simulink model "AQLRL"  (R2023b)
settings: Solver=FixedStepAuto  StartTime=0.0  StopTime=74.975  FixedStep=0.025  RelTol=1e-3
model workspace (MAT data in the model file):
  A = Simulink.Parameter
  A.Value = [1  0.025  0  0  0  0; 0  1  0  0  0  0; 0  0  1  0.025  0  0; 0  0  0  1  0  0; 0  0  0  0  1  0.025; 0  0  0  0  0  1]
  A.DataType = 'auto'
  A.Complexity = 'real'
  A.Dimensions = [6 6]
  Aag = Simulink.Parameter
  Aag.Value = [1  0.025  0  0  0  0; 0  1  0  0  0  0; 0  0  1  0.025  0  0; 0  0  0  1  0  0; 0  0  0  0  1  0.025; 0  0  0  0  0  1]
  Aag.DataType = 'auto'
  Aag.Complexity = 'real'
  Aag.Dimensions = [6 6]
  B = Simulink.Parameter
  B.Value = [-0.003065625  0  0; -0.24525  0  0; 0  0.003065625  0; 0  0.24525  0; 0  0  0.0003125; 0  0  0.025]
  B.DataType = 'auto'
  B.Complexity = 'real'
  B.Dimensions = [6 3]
  Bag = Simulink.Parameter
  Bag.Value = [0.0416666666667  0  0; 3.33333333333  0  0; 0  0.0416666666667  0; 0  3.33333333333  0; 0  0  0.0240384615385; 0  0  1.92307692308]
  Bag.DataType = 'auto'
  Bag.Complexity = 'real'
  Bag.Dimensions = [6 3]
  C = Simulink.Parameter
  C.Value = [1  0  0  0  0  0; 0  0  1  0  0  0; 0  0  0  0  1  0]
  C.DataType = 'auto'
  C.Complexity = 'real'
  C.Dimensions = [3 6]
  Cag = Simulink.Parameter
  Cag.Value = [1  0  0  0  0  0; 0  0  1  0  0  0; 0  0  0  0  1  0]
  Cag.DataType = 'auto'
  Cag.Complexity = 'real'
  Cag.Dimensions = [3 6]
  uang = [0 0 0 0 0 0 5.50670620214e-14 5.44009282066e-14 0 -3.99756362155e-05 -2.83106871279e-14 0 ... (9003 elements, 3x3001)]
  upos = [0 0 0 5.62466739851e-14 5.62327961973e-14 0 -2.39975660277e-05 4.94743135349e-14 0 -9.31686537426e-05 7.62168106405e-14 0 ... (9003 elements, 3x3001)]
values from neighbouring files (symbols this model uses):
  actions = [ ... (first row only)    [train_AQLRL.m]
  alpha = 0.5    [RL_iteration.m]    (also in RL_iteration2.m = 0.05; train_AQLRL.m = max(alpha * alpha_decay, alpha_min))
  epsilon = 0.4    [RL_iteration2.m]    (also in train_AQLRL.m = max(epsilon*epsilon_decay, epsilon_min))
  gamma = 0.9    [RL_iteration.m]    (also in RL_iteration2.m; train_AQLRL.m = 0.5)
  ref = [0 0 1.5 -3.29206127203e-06 0.00314263790126 1.5 -1.31682306379e-05 0.00628526200819 1.5 -2.96284647472e-05 0.00942785852649 1.5 ... (9000 elements, 3x3000)]    [circulartrajectory.mat]    (also in generate_circ_trajectory.m = [x;y;z]; generate_sprial_trajectory.m = [x;y;z]; generate_triangle_trajectory.m = [x;y;z]; spiralTrajectory.mat = [0 0 1.5 -2.96284647472e-05 0.00942785852649 1.50050016672 -)
  weights = evalin('base', 'weights')    [train_AQLRL.m]    (also in weights.mat = [0 0 0 0 0 0 0 0 0 0 0 0 ... (45 elements, 9x5)])
libraries: aerolibanimutils x1
(part 1 of 2)
settings Model: Creator=Lingf  LastModifiedBy=deandre
settings SolverCC: AlgebraicLoopSolver=TrustRegion
settings DataIOCC: ReturnWorkspaceOutputs=off
settings DebuggingCC: UnconnectedInputMsg=warning  UnconnectedOutputMsg=warning  UnconnectedLineMsg=warning  UnderSpecifiedDimensionMsg=warning
settings ModelReferenceCC: EnableRefExpFcnMdlSchedulingChecks=on
settings RTWCC: DLArmComputeVersion=19.05

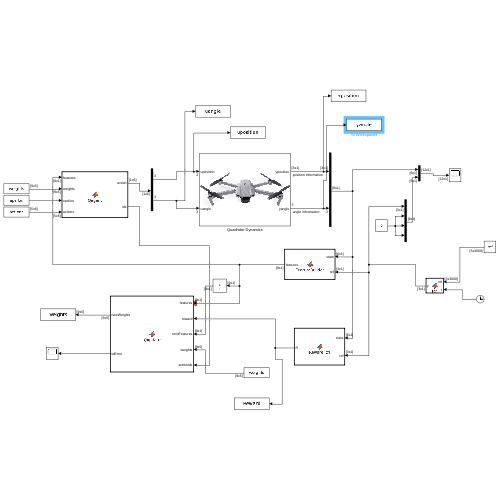
[thumbnail: Simulink's stored preview of the top-level diagram]
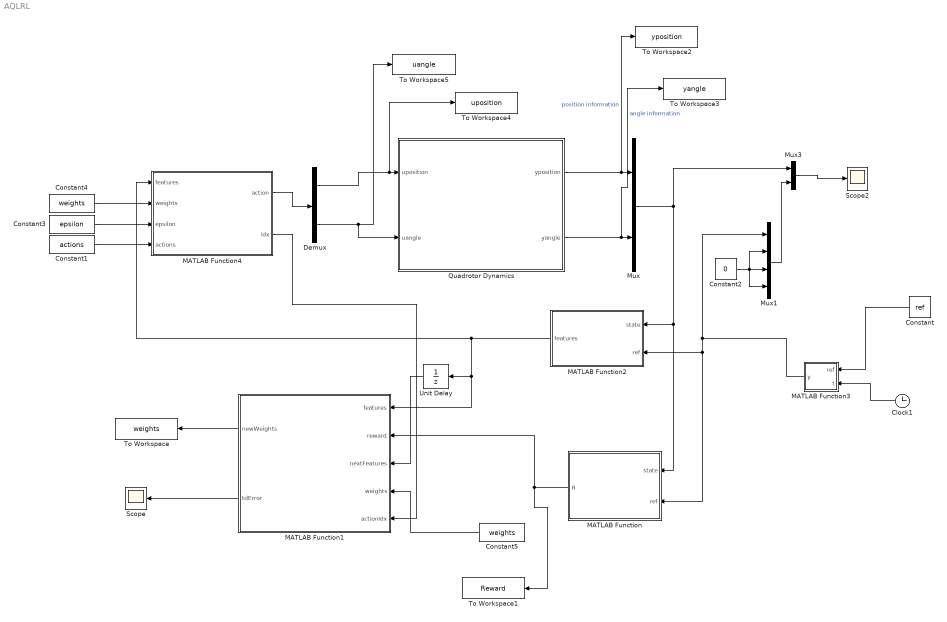
== system AQLRL ==
  Clock1 : Clock
  Constant : Constant  Value=ref
  Constant1 : Constant  Value=actions
  Constant2 : Constant  Value=0
  Constant3 : Constant  Value=epsilon
  Constant4 : Constant  Value=weights
  Constant5 : Constant  Value=weights
  Demux : Demux  Outputs=2
  MATLAB Function : MATLAB Function  TreatAsAtomicUnit=on
  MATLAB Function1 : MATLAB Function  TreatAsAtomicUnit=on
  MATLAB Function2 : MATLAB Function  TreatAsAtomicUnit=on
  MATLAB Function3 : MATLAB Function  TreatAsAtomicUnit=on
  MATLAB Function4 : MATLAB Function  TreatAsAtomicUnit=on
  Mux : Mux  Inputs=2
  Mux1 : Mux
  Mux3 : Mux  Inputs=2
  Quadrotor Dynamics : Subsystem
      mask Display: image('$imagefile'); % Use "Edit Image" on toolstrip to change.
  Scope : Scope
  Scope2 : Scope
  To Workspace : ToWorkspace  VariableName=weights  SampleTime=-1
      settings: Save2DSignal=2-D array (concatenate along first dimension)
  To Workspace1 : ToWorkspace  VariableName=Reward  SaveFormat=Structure With Time  SampleTime=-1
  To Workspace2 : ToWorkspace  VariableName=yposition  SaveFormat=Timeseries  SampleTime=-1
  To Workspace3 : ToWorkspace  VariableName=yangle  SaveFormat=Timeseries  SampleTime=-1
  To Workspace4 : ToWorkspace  VariableName=uposition  SaveFormat=Timeseries  SampleTime=-1
  To Workspace5 : ToWorkspace  VariableName=uangle  SaveFormat=Timeseries  SampleTime=-1
  Unit Delay : UnitDelay  SampleTime=-1  HasFrameUpgradeWarning=on
  wires:
  Quadrotor Dynamics/2(yangle) -> To Workspace3/1, Mux/2  "angle information"
  Quadrotor Dynamics/1(yposition) -> To Workspace2/1, Mux/1  "position information"
  Mux/1 -> Mux3/1, MATLAB Function2/1(state), MATLAB Function/1(state)
  Clock1/1 -> MATLAB Function3/2(t)
  Constant/1 -> MATLAB Function3/1(ref)
  MATLAB Function3/1(y) -> Mux1/1, MATLAB Function2/2(ref), MATLAB Function/2(ref)
  Mux3/1 -> Scope2/1
  MATLAB Function/1(R) -> To Workspace1/1, MATLAB Function1/2(reward)
  Constant5/1 -> MATLAB Function1/4(weights)
  MATLAB Function2/1(features) -> MATLAB Function4/1(features), Unit Delay/1, MATLAB Function1/1(features)
  Unit Delay/1 -> MATLAB Function1/3(nextFeatures)
  MATLAB Function1/1(newWeights) -> To Workspace/1
  MATLAB Function1/2(tdError) -> Scope/1
  Constant4/1 -> MATLAB Function4/2(weights)
  Constant3/1 -> MATLAB Function4/3(epsilon)
  Constant1/1 -> MATLAB Function4/4(actions)
  MATLAB Function4/1(action) -> Demux/1
  Demux/1 -> To Workspace4/1, Quadrotor Dynamics/1(uposition)
  Demux/2 -> To Workspace5/1, Quadrotor Dynamics/2(uangle)
  Constant2/1 -> Mux1/4, Mux1/3, Mux1/2
  Mux1/1 -> Mux3/2
  MATLAB Function4/2(idx) -> MATLAB Function1/5(actionIdx)
